simulink model "nlmpc_simulink"  (R2023a)
settings: Solver=VariableStepAuto  StartTime=0.0  StopTime=inf  RelTol=1e-3
settings Model: Creator=pindiche  LastModifiedBy=pindiche

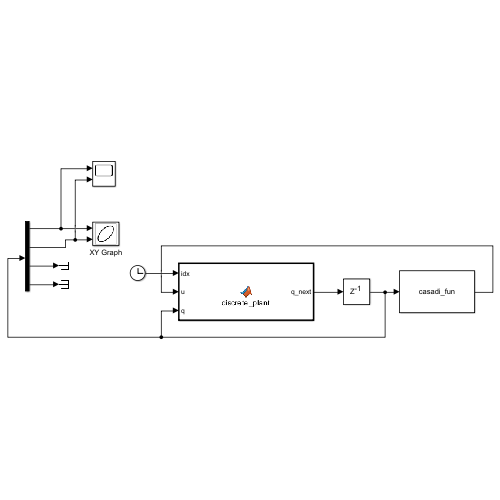
[thumbnail: Simulink's stored preview of the top-level diagram]
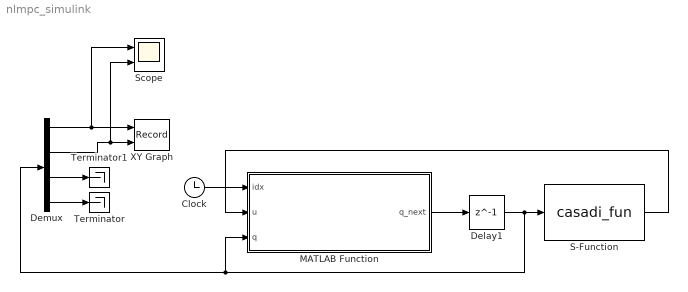
== system nlmpc_simulink ==
  Clock : Clock
  Delay1 : Delay  DelayLength=1  SampleTime=0.1
  Demux : Demux
  MATLAB Function : MATLAB Function  TreatAsAtomicUnit=on
  S-Function : S-Function  FunctionName=casadi_fun  Parameters='mpc_fun.casadi','mpc_fun'  SFunctionDeploymentMode=off  EnableBusSupport=off
  Scope : Scope  NumInputPorts=2
  Terminator : Terminator
  Terminator1 : Terminator
  XY Graph : Record  FileSettingsInternal="{\"entries\":[{\"content\":{\"excelSettings\":{\"content\":{},\"type\":\"Streamout.ExcelSettings\"}},\"type\":\"Streamout.FileSettingStorage\",\"uuid\":\"\"}],\"packageUris\":[\"http:\\/\\/schema.mathworks.com\\/mf0\\/streamout_blocks\\/R2020a\"],\"version\":\"1.0\"}"  Layout=[1 1]  SignalsInternal="{\"entries\":[{\"content\":{\"signals\":[{\"content\":{\"blockPath\":[],\"dimensions\":[1,1],\"domain\":\"\",\"lineColor\":\"#a2142f\",\"plots\":[1],\"port\":1,\"sid\":[\"\"],\"signalID\":15032,\"signalName\":\"Demux:1\"},\"type\":\"RecordBlkView.Signal\",\"uuid\":\"\"},{\"content\":{\"blockPath\":[],\"dimensions\":[1,1],\"domain\":\"\",\"lineColor\":\"#139fff\",\"plots\":[1],\"port\":2,\"sid\":[\"\"],\"signalID\":15036,\"signalName\":\"Demux:2\"},\"type\":\"RecordBlkView.Signal\",\"uuid\":\"\"}]},\"type\":\"RecordBlkView.InputSignals\",\"uuid\":\"\"}],\"packageUris\":[\"http:\\/\\/schema.mathworks.com\\/mf0\\/streamout_blocks\\/R2020a\"],\"version\":\"1.0\"}"  VisualizationBindings="{\"xyplotplugin\":{\"info\":[{\"series\":[{\"bindingParametersList\":[{\"parameter\":\"X-Axis\",\"signalID\":15032,\"signalName\":\"Demux:1\"},{\"parameter\":\"Y-Axis\",\"signalID\":15036,\"signalName\":\"Demux:2\"}],\"seriesID\":25840}],\"subplotID\":1}]}}"  CompatibilityTag=XY
  wires:
  S-Function/1 -> MATLAB Function/2(u)
  Demux/4 -> Terminator/1
  Demux/3 -> Terminator1/1
  Demux/1 -> XY Graph/1, Scope/1
  Demux/2 -> XY Graph/2, Scope/2
  Clock/1 -> MATLAB Function/1(idx)
  Delay1/1 -> MATLAB Function/3(q), Demux/1, S-Function/1
  MATLAB Function/1(q_next) -> Delay1/1

== matlab function nlmpc_simulink/MATLAB Function ==
  data: idx input; u input; q_next output; q input
function q_next = discrete_plant(idx, u, q)
    % Np = 12;
    % t = 0:0.1:100;
    % % Circle reference
    % alpha   = 5;
    % beta    = 5;
    % ang     = 0.2;
    % xr = alpha*cos(ang*t);      dxr = -alpha*ang*sin(ang*t);    ddxr = -alpha*ang*ang*cos(ang*t);       dddxr = alpha*ang*ang*ang*sin(ang*t);
    % yr = beta*sin(ang*t);       dyr = beta*ang*cos(ang*t);      ddyr = -beta*ang*ang*sin(ang*t);        dddyr = -beta*ang*ang*ang*cos(ang*t);
    % 
    % % % % % % % % % % % % % % % % % %
    % 
    % % Computing real input reference
    % Vr      = sqrt(dxr.*dxr + dyr.*dyr);
    % omegar  = l * Vr .* ((dddyr.*dxr - dddxr.*dyr).*Vr.*Vr - 3 * (ddyr.*dxr - ddxr.*dyr) .* (dxr.*ddxr + dyr.*ddyr)) ...
    %           ./ (Vr.^6 + l*l*(ddyr.*dxr - ddxr.*dyr).^2);
    % uref = [Vr; omegar];
    % 
    % % Computing angle reference
    % thetar  = unwrap(atan2(dyr ./ Vr, dxr ./ Vr));
    % phir    = atan((l*(ddyr.*dxr - ddxr.*dyr)) ./ Vr.^3);
    % 
    % xref = [xr; yr; thetar; phir];
    % 
    % xref = xref(:, idx:idx+Np);
    
    % Parameters
    l = 0.256;
    dt = 0.1;  
    x = q(1);
    y = q(2);
    theta = q(3);
    phi = q(4);
    
    % Extract control inputs
    v = u(1); 
    omega = u(2);  

    % Discretized system dynamics
    x_next = x + dt * (v * cos(theta));  
    y_next = y + dt * (v * sin(theta)); 
    theta_next = theta + dt * (v / l * tan(phi));  
    phi_next = phi + dt * omega; 

    q_next = [x_next; y_next; theta_next; phi_next];
end
